simulink model "V.1.0.SystemsmModelling"  (R2020a)
settings: Solver=ode23t  StartTime=0.0  StopTime=2000  MaxStep=2000.0  RelTol=1e-3
values from neighbouring files (symbols this model uses):
  InitialTemp = 300    [Setup.m]
undefined symbols (not defined in the file or in its folder): commanded_mass_flow, compressor_time_constant, condenser_length, copper_density, environment_temperature, evaporator_length, ground_temperature, max_throat_area, max_throat_temperature, min_throat_area, min_throat_temperature, pipe_diameter, pipe_thickness, target_temperature, temperature_delta, u_sat
libraries: fl_lib x208, refrigeration_lib x90, fl_ps_legacy_lib x50, nesl_utility x45
(part 5 of 7)

== system V.1.0.SystemsmModelling/Air Conditioning System/Air Conditioner Model5/Condenser ==
  Condenser Conduction : fl_lib/Thermal/Thermal Elements/Conductive Heat Transfer  area=pi*pipe_diameter*condenser_length m^2  thickness=pipe_thickness m  th_cond=copper_conductivity W/(m*K)  T_specify=off  T_priority=High  T=0 K  T_nominal_specify=off  T_nominal_unit=K  T_nominal_value=1  Q_specify=off  Q_priority=High  Q=0 J/s  Q_nominal_specify=off  Q_nominal_unit=W  Q_nominal_value=1
  Condenser Copper : fl_lib/Thermal/Thermal Elements/Thermal Mass  mass=pi*pipe_diameter*condenser_length*pipe_thickness*copper_density kg  sp_heat=copper_specific_heat J/kg/K  T_specify=on  T_priority=High  T=environment_temperature K  T_nominal_specify=off  T_nominal_unit=K  T_nominal_value=1  Q_specify=off  Q_priority=High  Q=0 J/s  Q_nominal_specify=off  Q_nominal_unit=W  Q_nominal_value=1
  Condenser Pipe : refrigeration_lib/Pipe  L=condenser_length m  S=pi*pipe_diameter^2/4 m^2  Dh=pipe_diameter m  fs=64  La=0.1*condenser_length m  eps=15e-6 m  Re_lam=2000  Re_tur=4000  J_smooth=5 kg/m^2/s  p_0=charge_pressure MPa  T_0=-1 K  x_0=initial_quality  mdot_A_specify=off  mdot_A_priority=High  mdot_A=0 kg/s  mdot_A_nominal_specify=off  mdot_A_nominal_unit=kg/s  mdot_A_nominal_value=1  mdot_B_specify=off  mdot_B_priority=High  mdot_B=0 kg/s  mdot_B_nominal_specify=off  mdot_B_nominal_unit=kg/s  mdot_B_nominal_value=1  phi_A_specify=off  phi_A_priority=High  phi_A=0 kW  phi_A_nominal_specify=off  phi_A_nominal_unit=kW  phi_A_nominal_value=1  phi_B_specify=off  phi_B_priority=High  phi_B=0 kW  phi_B_nominal_specify=off  phi_B_nominal_unit=kW  phi_B_nominal_value=1  v_A_specify=off  v_A_priority=High  v_A=0.230606289431 m^3/kg  v_A_nominal_specify=off  v_A_nominal_unit=m^3/kg  v_A_nominal_value=1  v_B_specify=off  v_B_priority=High  v_B=0.230606289431 m^3/kg  v_B_nominal_specify=off  v_B_nominal_unit=m^3/kg  v_B_nominal_value=1  p_I_specify=off  p_I_priority=High  p_I=0.101325 MPa  p_I_nominal_specify=off  p_I_nominal_unit=MPa  p_I_nominal_value=1  u_I_specify=off  u_I_priority=High  u_I=396.921741345 kJ/kg  u_I_nominal_specify=off  u_I_nominal_unit=kJ/kg  u_I_nominal_value=1  v_I_specify=off  v_I_priority=High  v_I=0.230606289431 m^3/kg  v_I_nominal_specify=off  v_I_nominal_unit=m^3/kg  v_I_nominal_value=1  q_T_specify=off  q_T_priority=High  q_T=0 kW  q_T_nominal_specify=off  q_T_nominal_unit=kW  q_T_nominal_value=1  Ff_A_specify=off  Ff_A_priority=High  Ff_A=0 N  Ff_A_nominal_specify=off  Ff_A_nominal_unit=N  Ff_A_nominal_value=1  Ff_B_specify=off  Ff_B_priority=High  Ff_B=0 N  Ff_B_nominal_specify=off  Ff_B_nominal_unit=N  Ff_B_nominal_value=1  ev_I_specify=off  ev_I_priority=High  ev_I=1.7212095226213e+3 kJ/m^3  ev_I_nominal_specify=off  ev_I_nominal_unit=kJ/m^3  ev_I_nominal_value=1  mdot_I_specify=off  mdot_I_priority=High  mdot_I=0 kg/s  mdot_I_nominal_specify=off  mdot_I_nominal_unit=kg/s  mdot_I_nominal_value=1  Nu_I_specify=off  Nu_I_priority=High  Nu_I=0  Nu_I_nominal_specify=off  Nu_I_nominal_unit=1  Nu_I_nominal_value=1
      settings: InternalSimscapePortConfiguration="{\"Bottom\":[],\"Left\":[{\"id\":\"A\",\"label\":\"A\",\"type\":\"refrigeration.refrigeration\"},{\"id\":\"T\",\"label\":\"T\",\"type\":\"foundation.thermal.thermal\"}],\"Right\":[{\"id\":\"B\",\"label\":\"B\",\"type\":\"refrigeration.refrigeration\"}],\"Top\":[]}"
  T : PMIOPort  Side=Left
  B : PMIOPort  Port=2  Side=Left
  A : PMIOPort  Port=3  Side=Right
  connections:
  Condenser Conduction/LConn1 -- Condenser Pipe/LConn2 -- Condenser Copper/LConn1
  T/RConn1 -- Condenser Conduction/RConn1
  B/RConn1 -- Condenser Pipe/RConn1
  Condenser Pipe/LConn1 -- A/RConn1

== system V.1.0.SystemsmModelling/Air Conditioning System/Air Conditioner Model5/Control ==
  Err : Inport
  Relay : Relay  OnSwitchValue=temperature_delta  OffSwitchValue=-temperature_delta
  On : Outport
  wires:
  Err/1 -> Relay/1
  Relay/1 -> On/1

== system V.1.0.SystemsmModelling/Air Conditioning System/Air Conditioner Model5/Environment ==
  Condenser Convection : fl_lib/Thermal/Thermal Elements/Convective Heat Transfer  area=fin_area m^2  heat_tr_coeff=fin_convection_coefficient W/(m^2 * K)  T_specify=off  T_priority=High  T=0 K  T_nominal_specify=off  T_nominal_unit=K  T_nominal_value=1  Q_specify=off  Q_priority=High  Q=0 J/s  Q_nominal_specify=off  Q_nominal_unit=W  Q_nominal_value=1
  Constant : Constant  Value=environment_temperature
  Ideal Temperature Source : fl_lib/Thermal/Thermal Sources/Controlled Temperature Source
  Simulink-PS Converter : nesl_utility/Simulink-PS Converter  PhysicalDomain=network_engine_domain  SubClassName=ps_input  LeftPortType=input  RightPortType=output  PseudoPeriodic=off  Frequencies=[]  NoiseDistribution=none  NoiseParameters=[]  Unit=K  AffineConversion=off  FilteringAndDerivatives=zero  SimscapeFilterOrder=1  InputFilterTimeConstant=0.001  UdotUserProvided=1
  Thermal Reference : fl_lib/Thermal/Thermal Elements/Thermal Reference
  T : PMIOPort  Side=Left
  wires:
  Constant/1 -> Simulink-PS Converter/1
  connections:
  Condenser Convection/RConn1 -- Ideal Temperature Source/LConn1
  Condenser Convection/LConn1 -- T/RConn1
  Ideal Temperature Source/RConn1 -- Simulink-PS Converter/RConn1
  Ideal Temperature Source/RConn2 -- Thermal Reference/LConn1

== system V.1.0.SystemsmModelling/Air Conditioning System/Air Conditioner Model5/Evaporator ==
  Evaporator Conduction : fl_lib/Thermal/Thermal Elements/Conductive Heat Transfer  area=pi*pipe_diameter*evaporator_length m^2  thickness=pipe_thickness m  th_cond=copper_conductivity W/(m*K)  T_specify=off  T_priority=High  T=0 K  T_nominal_specify=off  T_nominal_unit=K  T_nominal_value=1  Q_specify=off  Q_priority=High  Q=0 J/s  Q_nominal_specify=off  Q_nominal_unit=W  Q_nominal_value=1
  Evaporator Copper : fl_lib/Thermal/Thermal Elements/Thermal Mass  mass=pi*pipe_diameter*evaporator_length*pipe_thickness*copper_density kg  sp_heat=copper_specific_heat J/kg/K  T_specify=on  T_priority=High  T=target_temperature K  T_nominal_specify=off  T_nominal_unit=K  T_nominal_value=1  Q_specify=off  Q_priority=High  Q=0 J/s  Q_nominal_specify=off  Q_nominal_unit=W  Q_nominal_value=1
  Evaporator Pipe : refrigeration_lib/Pipe  L=evaporator_length m  S=pi*pipe_diameter^2/4 m^2  Dh=pipe_diameter m  fs=64  La=0.1*evaporator_length m  eps=15e-6 m  Re_lam=2000  Re_tur=4000  J_smooth=5 kg/m^2/s  p_0=charge_pressure MPa  T_0=-1 K  x_0=initial_quality  mdot_A_specify=off  mdot_A_priority=High  mdot_A=0 kg/s  mdot_A_nominal_specify=off  mdot_A_nominal_unit=kg/s  mdot_A_nominal_value=1  mdot_B_specify=off  mdot_B_priority=High  mdot_B=0 kg/s  mdot_B_nominal_specify=off  mdot_B_nominal_unit=kg/s  mdot_B_nominal_value=1  phi_A_specify=off  phi_A_priority=High  phi_A=0 kW  phi_A_nominal_specify=off  phi_A_nominal_unit=kW  phi_A_nominal_value=1  phi_B_specify=off  phi_B_priority=High  phi_B=0 kW  phi_B_nominal_specify=off  phi_B_nominal_unit=kW  phi_B_nominal_value=1  v_A_specify=off  v_A_priority=High  v_A=0.230606289431 m^3/kg  v_A_nominal_specify=off  v_A_nominal_unit=m^3/kg  v_A_nominal_value=1  v_B_specify=off  v_B_priority=High  v_B=0.230606289431 m^3/kg  v_B_nominal_specify=off  v_B_nominal_unit=m^3/kg  v_B_nominal_value=1  p_I_specify=off  p_I_priority=High  p_I=0.101325 MPa  p_I_nominal_specify=off  p_I_nominal_unit=MPa  p_I_nominal_value=1  u_I_specify=off  u_I_priority=High  u_I=396.921741345 kJ/kg  u_I_nominal_specify=off  u_I_nominal_unit=kJ/kg  u_I_nominal_value=1  v_I_specify=off  v_I_priority=High  v_I=0.230606289431 m^3/kg  v_I_nominal_specify=off  v_I_nominal_unit=m^3/kg  v_I_nominal_value=1  q_T_specify=off  q_T_priority=High  q_T=0 kW  q_T_nominal_specify=off  q_T_nominal_unit=kW  q_T_nominal_value=1  Ff_A_specify=off  Ff_A_priority=High  Ff_A=0 N  Ff_A_nominal_specify=off  Ff_A_nominal_unit=N  Ff_A_nominal_value=1  Ff_B_specify=off  Ff_B_priority=High  Ff_B=0 N  Ff_B_nominal_specify=off  Ff_B_nominal_unit=N  Ff_B_nominal_value=1  ev_I_specify=off  ev_I_priority=High  ev_I=1.7212095226213e+3 kJ/m^3  ev_I_nominal_specify=off  ev_I_nominal_unit=kJ/m^3  ev_I_nominal_value=1  mdot_I_specify=off  mdot_I_priority=High  mdot_I=0 kg/s  mdot_I_nominal_specify=off  mdot_I_nominal_unit=kg/s  mdot_I_nominal_value=1  Nu_I_specify=off  Nu_I_priority=High  Nu_I=0  Nu_I_nominal_specify=off  Nu_I_nominal_unit=1  Nu_I_nominal_value=1
      settings: InternalSimscapePortConfiguration="{\"Bottom\":[],\"Left\":[{\"id\":\"A\",\"label\":\"A\",\"type\":\"refrigeration.refrigeration\"},{\"id\":\"T\",\"label\":\"T\",\"type\":\"foundation.thermal.thermal\"}],\"Right\":[{\"id\":\"B\",\"label\":\"B\",\"type\":\"refrigeration.refrigeration\"}],\"Top\":[]}"
  A : PMIOPort  Side=Left
  B : PMIOPort  Port=2  Side=Right
  T : PMIOPort  Port=3  Side=Right
  connections:
  Evaporator Conduction/RConn1 -- T/RConn1
  Evaporator Copper/LConn1 -- Evaporator Pipe/LConn2 -- Evaporator Conduction/LConn1
  Evaporator Pipe/RConn1 -- B/RConn1
  Evaporator Pipe/LConn1 -- A/RConn1

== system V.1.0.SystemsmModelling/Air Conditioning System/Air Conditioner Model5/Expansion Valve ==
  Controlled Local Restriction : refrigeration_lib/Controlled Local Restriction  Cd=0.7  L=0.1 m  S=pi*pipe_diameter^2/4 m^2
      settings: InternalSimscapePortConfiguration="{\"Bottom\":[],\"Left\":[{\"id\":\"A\",\"label\":\"A\",\"type\":\"refrigeration.refrigeration\"},{\"id\":\"Sr\",\"label\":\"S\",\"type\":\"input\"}],\"Right\":[{\"id\":\"B\",\"label\":\"B\",\"type\":\"refrigeration.refrigeration\"}],\"Top\":[]}"
  Cycle Sensor 4 : Subsystem
  Mass Flow Sensor : Subsystem
  Valve Control : Subsystem
  A : PMIOPort  Side=Left
  B : PMIOPort  Port=2  Side=Right
  connections:
  B/RConn1 -- Cycle Sensor 4/LConn1 -- Mass Flow Sensor/RConn1
  Controlled Local Restriction/LConn1 -- A/RConn1
  Controlled Local Restriction/RConn1 -- Mass Flow Sensor/LConn1
  Controlled Local Restriction/LConn2 -- Valve Control/LConn1
  Cycle Sensor 4/RConn1 -- Valve Control/RConn1

== system V.1.0.SystemsmModelling/Air Conditioning System/Air Conditioner Model5/Plot Properties ==

== system V.1.0.SystemsmModelling/Air Conditioning System/Air Conditioner Model5/Refrigerator Compartment ==
  Environment Temperature : Subsystem
  Evaporator Convection : fl_lib/Thermal/Thermal Elements/Convective Heat Transfer  area=interior_surface_area m^2  heat_tr_coeff=natural_convection_coefficient W/(m^2 * K)  T_specify=off  T_priority=High  T=0 K  T_nominal_specify=off  T_nominal_unit=K  T_nominal_value=1  Q_specify=off  Q_priority=High  Q=0 J/s  Q_nominal_specify=off  Q_nominal_unit=W  Q_nominal_value=1
  Heat Flow Sensor : Subsystem
  Polyurethane Foam Conduction : fl_lib/Thermal/Thermal Elements/Conductive Heat Transfer  area=interior_surface_area m^2  thickness=foam_thickness m  th_cond=foam_conductivity W/(m*K)  T_specify=off  T_priority=High  T=0 K  T_nominal_specify=off  T_nominal_unit=K  T_nominal_value=1  Q_specify=off  Q_priority=High  Q=0 J/s  Q_nominal_specify=off  Q_nominal_unit=W  Q_nominal_value=1
  Refrigerator Convection Exterior : fl_lib/Thermal/Thermal Elements/Convective Heat Transfer  area=exterior_surface_area m^2  heat_tr_coeff=natural_convection_coefficient W/(m^2 * K)  T_specify=off  T_priority=High  T=0 K  T_nominal_specify=off  T_nominal_unit=K  T_nominal_value=1  Q_specify=off  Q_priority=High  Q=0 J/s  Q_nominal_specify=off  Q_nominal_unit=W  Q_nominal_value=1
  Refrigerator Convection Interior : fl_lib/Thermal/Thermal Elements/Convective Heat Transfer  area=interior_surface_area m^2  heat_tr_coeff=natural_convection_coefficient W/(m^2 * K)  T_specify=off  T_priority=High  T=0 K  T_nominal_specify=off  T_nominal_unit=K  T_nominal_value=1  Q_specify=off  Q_priority=High  Q=0 J/s  Q_nominal_specify=off  Q_nominal_unit=W  Q_nominal_value=1
  Temperature Sensor : Subsystem
  T : PMIOPort  Side=Left
  Air : PMIOPort  Port=2  Side=Left
  S : Outport
  wires:
  Temperature Sensor/1(T) -> S/1
  connections:
  Evaporator Convection/LConn1 -- Heat Flow Sensor/RConn1
  T/RConn1 -- Heat Flow Sensor/LConn1
  Refrigerator Convection Exterior/RConn1 -- Environment Temperature/LConn1
  Refrigerator Convection Interior/LConn1 -- Evaporator Convection/RConn1 -- Temperature Sensor/LConn1 -- Air/RConn1
  Refrigerator Convection Interior/RConn1 -- Polyurethane Foam Conduction/LConn1
  Polyurethane Foam Conduction/RConn1 -- Refrigerator Convection Exterior/LConn1

== system V.1.0.SystemsmModelling/Air Conditioning System/Air Conditioner Model6/Compressor ==
  On : Inport
  Commanded Mass Flow Rate : Gain  Gain=commanded_mass_flow
  Compressor Lag : TransferFcn  Numerator=[(9/compressor_time_constant)^2]  Denominator=[1, 2*(9/compressor_time_constant), (9/compressor_time_constant)^2]
  Controlled Mass Flow Rate Source : refrigeration_lib/Controlled Mass Flow Rate Source  S=pi*pipe_diameter^2/4 m^2  L=0.1 m  mdot_specify=off  mdot_priority=High  mdot=0 kg/s  mdot_nominal_specify=off  mdot_nominal_unit=kg/s  mdot_nominal_value=1  phi_A_specify=off  phi_A_priority=High  phi_A=0 kW  phi_A_nominal_specify=off  phi_A_nominal_unit=kW  phi_A_nominal_value=1  phi_B_specify=off  phi_B_priority=High  phi_B=0 kW  phi_B_nominal_specify=off  phi_B_nominal_unit=kW  phi_B_nominal_value=1  u_AI_specify=off  u_AI_priority=High  u_AI=396.921741345 kJ/kg  u_AI_nominal_specify=off  u_AI_nominal_unit=kJ/kg  u_AI_nominal_value=1  v_A_specify=off  v_A_priority=High  v_A=0.230606289431 m^3/kg  v_A_nominal_specify=off  v_A_nominal_unit=m^3/kg  v_A_nominal_value=1  u_BI_specify=off  u_BI_priority=High  u_BI=396.921741345 kJ/kg  u_BI_nominal_specify=off  u_BI_nominal_unit=kJ/kg  u_BI_nominal_value=1  v_B_specify=off  v_B_priority=High  v_B=0.230606289431 m^3/kg  v_B_nominal_specify=off  v_B_nominal_unit=m^3/kg  v_B_nominal_value=1  u_2_specify=off  u_2_priority=High  u_2=396.921741345 kJ/kg  u_2_nominal_specify=off  u_2_nominal_unit=kJ/kg  u_2_nominal_value=1  u_3_specify=off  u_3_priority=High  u_3=396.921741345 kJ/kg  u_3_nominal_specify=off  u_3_nominal_unit=kJ/kg  u_3_nominal_value=1
      settings: InternalSimscapePortConfiguration="{\"Bottom\":[],\"Left\":[{\"id\":\"A\",\"label\":\"A\",\"type\":\"refrigeration.refrigeration\"},{\"id\":\"M\",\"label\":\"M\",\"type\":\"input\"}],\"Right\":[{\"id\":\"B\",\"label\":\"B\",\"type\":\"refrigeration.refrigeration\"},{\"id\":\"W\",\"label\":\"W\",\"type\":\"output\"}],\"Top\":[]}"
  Simulink-PS Converter : nesl_utility/Simulink-PS Converter  PhysicalDomain=network_engine_domain  SubClassName=ps_input  LeftPortType=input  RightPortType=output  PseudoPeriodic=off  Frequencies=[]  NoiseDistribution=none  NoiseParameters=[]  Unit=kg/s  AffineConversion=off  FilteringAndDerivatives=zero  SimscapeFilterOrder=1  InputFilterTimeConstant=0.001  UdotUserProvided=1
  B : PMIOPort  Side=Right
  A : PMIOPort  Port=2  Side=Left
  wires:
  Compressor Lag/1 -> Simulink-PS Converter/1
  Commanded Mass Flow Rate/1 -> Compressor Lag/1
  On/1 -> Commanded Mass Flow Rate/1
  connections:
  Controlled Mass Flow Rate Source/RConn1 -- B/RConn1
  Controlled Mass Flow Rate Source/LConn2 -- Simulink-PS Converter/RConn1
  A/RConn1 -- Controlled Mass Flow Rate Source/LConn1

== system V.1.0.SystemsmModelling/Air Conditioning System/Air Conditioner Model6/Condenser ==
  Condenser Conduction : fl_lib/Thermal/Thermal Elements/Conductive Heat Transfer  area=pi*pipe_diameter*condenser_length m^2  thickness=pipe_thickness m  th_cond=copper_conductivity W/(m*K)  T_specify=off  T_priority=High  T=0 K  T_nominal_specify=off  T_nominal_unit=K  T_nominal_value=1  Q_specify=off  Q_priority=High  Q=0 J/s  Q_nominal_specify=off  Q_nominal_unit=W  Q_nominal_value=1
  Condenser Copper : fl_lib/Thermal/Thermal Elements/Thermal Mass  mass=pi*pipe_diameter*condenser_length*pipe_thickness*copper_density kg  sp_heat=copper_specific_heat J/kg/K  T_specify=on  T_priority=High  T=environment_temperature K  T_nominal_specify=off  T_nominal_unit=K  T_nominal_value=1  Q_specify=off  Q_priority=High  Q=0 J/s  Q_nominal_specify=off  Q_nominal_unit=W  Q_nominal_value=1
  Condenser Pipe : refrigeration_lib/Pipe  L=condenser_length m  S=pi*pipe_diameter^2/4 m^2  Dh=pipe_diameter m  fs=64  La=0.1*condenser_length m  eps=15e-6 m  Re_lam=2000  Re_tur=4000  J_smooth=5 kg/m^2/s  p_0=charge_pressure MPa  T_0=-1 K  x_0=initial_quality  mdot_A_specify=off  mdot_A_priority=High  mdot_A=0 kg/s  mdot_A_nominal_specify=off  mdot_A_nominal_unit=kg/s  mdot_A_nominal_value=1  mdot_B_specify=off  mdot_B_priority=High  mdot_B=0 kg/s  mdot_B_nominal_specify=off  mdot_B_nominal_unit=kg/s  mdot_B_nominal_value=1  phi_A_specify=off  phi_A_priority=High  phi_A=0 kW  phi_A_nominal_specify=off  phi_A_nominal_unit=kW  phi_A_nominal_value=1  phi_B_specify=off  phi_B_priority=High  phi_B=0 kW  phi_B_nominal_specify=off  phi_B_nominal_unit=kW  phi_B_nominal_value=1  v_A_specify=off  v_A_priority=High  v_A=0.230606289431 m^3/kg  v_A_nominal_specify=off  v_A_nominal_unit=m^3/kg  v_A_nominal_value=1  v_B_specify=off  v_B_priority=High  v_B=0.230606289431 m^3/kg  v_B_nominal_specify=off  v_B_nominal_unit=m^3/kg  v_B_nominal_value=1  p_I_specify=off  p_I_priority=High  p_I=0.101325 MPa  p_I_nominal_specify=off  p_I_nominal_unit=MPa  p_I_nominal_value=1  u_I_specify=off  u_I_priority=High  u_I=396.921741345 kJ/kg  u_I_nominal_specify=off  u_I_nominal_unit=kJ/kg  u_I_nominal_value=1  v_I_specify=off  v_I_priority=High  v_I=0.230606289431 m^3/kg  v_I_nominal_specify=off  v_I_nominal_unit=m^3/kg  v_I_nominal_value=1  q_T_specify=off  q_T_priority=High  q_T=0 kW  q_T_nominal_specify=off  q_T_nominal_unit=kW  q_T_nominal_value=1  Ff_A_specify=off  Ff_A_priority=High  Ff_A=0 N  Ff_A_nominal_specify=off  Ff_A_nominal_unit=N  Ff_A_nominal_value=1  Ff_B_specify=off  Ff_B_priority=High  Ff_B=0 N  Ff_B_nominal_specify=off  Ff_B_nominal_unit=N  Ff_B_nominal_value=1  ev_I_specify=off  ev_I_priority=High  ev_I=1.7212095226213e+3 kJ/m^3  ev_I_nominal_specify=off  ev_I_nominal_unit=kJ/m^3  ev_I_nominal_value=1  mdot_I_specify=off  mdot_I_priority=High  mdot_I=0 kg/s  mdot_I_nominal_specify=off  mdot_I_nominal_unit=kg/s  mdot_I_nominal_value=1  Nu_I_specify=off  Nu_I_priority=High  Nu_I=0  Nu_I_nominal_specify=off  Nu_I_nominal_unit=1  Nu_I_nominal_value=1
      settings: InternalSimscapePortConfiguration="{\"Bottom\":[],\"Left\":[{\"id\":\"A\",\"label\":\"A\",\"type\":\"refrigeration.refrigeration\"},{\"id\":\"T\",\"label\":\"T\",\"type\":\"foundation.thermal.thermal\"}],\"Right\":[{\"id\":\"B\",\"label\":\"B\",\"type\":\"refrigeration.refrigeration\"}],\"Top\":[]}"
  T : PMIOPort  Side=Left
  B : PMIOPort  Port=2  Side=Left
  A : PMIOPort  Port=3  Side=Right
  connections:
  Condenser Conduction/LConn1 -- Condenser Pipe/LConn2 -- Condenser Copper/LConn1
  T/RConn1 -- Condenser Conduction/RConn1
  B/RConn1 -- Condenser Pipe/RConn1
  Condenser Pipe/LConn1 -- A/RConn1

== system V.1.0.SystemsmModelling/Air Conditioning System/Air Conditioner Model6/Control ==
  Err : Inport
  Relay : Relay  OnSwitchValue=temperature_delta  OffSwitchValue=-temperature_delta
  On : Outport
  wires:
  Err/1 -> Relay/1
  Relay/1 -> On/1

== system V.1.0.SystemsmModelling/Air Conditioning System/Air Conditioner Model6/Environment ==
  Condenser Convection : fl_lib/Thermal/Thermal Elements/Convective Heat Transfer  area=fin_area m^2  heat_tr_coeff=fin_convection_coefficient W/(m^2 * K)  T_specify=off  T_priority=High  T=0 K  T_nominal_specify=off  T_nominal_unit=K  T_nominal_value=1  Q_specify=off  Q_priority=High  Q=0 J/s  Q_nominal_specify=off  Q_nominal_unit=W  Q_nominal_value=1
  Constant : Constant  Value=environment_temperature
  Ideal Temperature Source : fl_lib/Thermal/Thermal Sources/Controlled Temperature Source
  Simulink-PS Converter : nesl_utility/Simulink-PS Converter  PhysicalDomain=network_engine_domain  SubClassName=ps_input  LeftPortType=input  RightPortType=output  PseudoPeriodic=off  Frequencies=[]  NoiseDistribution=none  NoiseParameters=[]  Unit=K  AffineConversion=off  FilteringAndDerivatives=zero  SimscapeFilterOrder=1  InputFilterTimeConstant=0.001  UdotUserProvided=1
  Thermal Reference : fl_lib/Thermal/Thermal Elements/Thermal Reference
  T : PMIOPort  Side=Left
  wires:
  Constant/1 -> Simulink-PS Converter/1
  connections:
  Condenser Convection/RConn1 -- Ideal Temperature Source/LConn1
  Condenser Convection/LConn1 -- T/RConn1
  Ideal Temperature Source/RConn1 -- Simulink-PS Converter/RConn1
  Ideal Temperature Source/RConn2 -- Thermal Reference/LConn1

== system V.1.0.SystemsmModelling/Air Conditioning System/Air Conditioner Model6/Evaporator ==
  Evaporator Conduction : fl_lib/Thermal/Thermal Elements/Conductive Heat Transfer  area=pi*pipe_diameter*evaporator_length m^2  thickness=pipe_thickness m  th_cond=copper_conductivity W/(m*K)  T_specify=off  T_priority=High  T=0 K  T_nominal_specify=off  T_nominal_unit=K  T_nominal_value=1  Q_specify=off  Q_priority=High  Q=0 J/s  Q_nominal_specify=off  Q_nominal_unit=W  Q_nominal_value=1
  Evaporator Copper : fl_lib/Thermal/Thermal Elements/Thermal Mass  mass=pi*pipe_diameter*evaporator_length*pipe_thickness*copper_density kg  sp_heat=copper_specific_heat J/kg/K  T_specify=on  T_priority=High  T=target_temperature K  T_nominal_specify=off  T_nominal_unit=K  T_nominal_value=1  Q_specify=off  Q_priority=High  Q=0 J/s  Q_nominal_specify=off  Q_nominal_unit=W  Q_nominal_value=1
  Evaporator Pipe : refrigeration_lib/Pipe  L=evaporator_length m  S=pi*pipe_diameter^2/4 m^2  Dh=pipe_diameter m  fs=64  La=0.1*evaporator_length m  eps=15e-6 m  Re_lam=2000  Re_tur=4000  J_smooth=5 kg/m^2/s  p_0=charge_pressure MPa  T_0=-1 K  x_0=initial_quality  mdot_A_specify=off  mdot_A_priority=High  mdot_A=0 kg/s  mdot_A_nominal_specify=off  mdot_A_nominal_unit=kg/s  mdot_A_nominal_value=1  mdot_B_specify=off  mdot_B_priority=High  mdot_B=0 kg/s  mdot_B_nominal_specify=off  mdot_B_nominal_unit=kg/s  mdot_B_nominal_value=1  phi_A_specify=off  phi_A_priority=High  phi_A=0 kW  phi_A_nominal_specify=off  phi_A_nominal_unit=kW  phi_A_nominal_value=1  phi_B_specify=off  phi_B_priority=High  phi_B=0 kW  phi_B_nominal_specify=off  phi_B_nominal_unit=kW  phi_B_nominal_value=1  v_A_specify=off  v_A_priority=High  v_A=0.230606289431 m^3/kg  v_A_nominal_specify=off  v_A_nominal_unit=m^3/kg  v_A_nominal_value=1  v_B_specify=off  v_B_priority=High  v_B=0.230606289431 m^3/kg  v_B_nominal_specify=off  v_B_nominal_unit=m^3/kg  v_B_nominal_value=1  p_I_specify=off  p_I_priority=High  p_I=0.101325 MPa  p_I_nominal_specify=off  p_I_nominal_unit=MPa  p_I_nominal_value=1  u_I_specify=off  u_I_priority=High  u_I=396.921741345 kJ/kg  u_I_nominal_specify=off  u_I_nominal_unit=kJ/kg  u_I_nominal_value=1  v_I_specify=off  v_I_priority=High  v_I=0.230606289431 m^3/kg  v_I_nominal_specify=off  v_I_nominal_unit=m^3/kg  v_I_nominal_value=1  q_T_specify=off  q_T_priority=High  q_T=0 kW  q_T_nominal_specify=off  q_T_nominal_unit=kW  q_T_nominal_value=1  Ff_A_specify=off  Ff_A_priority=High  Ff_A=0 N  Ff_A_nominal_specify=off  Ff_A_nominal_unit=N  Ff_A_nominal_value=1  Ff_B_specify=off  Ff_B_priority=High  Ff_B=0 N  Ff_B_nominal_specify=off  Ff_B_nominal_unit=N  Ff_B_nominal_value=1  ev_I_specify=off  ev_I_priority=High  ev_I=1.7212095226213e+3 kJ/m^3  ev_I_nominal_specify=off  ev_I_nominal_unit=kJ/m^3  ev_I_nominal_value=1  mdot_I_specify=off  mdot_I_priority=High  mdot_I=0 kg/s  mdot_I_nominal_specify=off  mdot_I_nominal_unit=kg/s  mdot_I_nominal_value=1  Nu_I_specify=off  Nu_I_priority=High  Nu_I=0  Nu_I_nominal_specify=off  Nu_I_nominal_unit=1  Nu_I_nominal_value=1
      settings: InternalSimscapePortConfiguration="{\"Bottom\":[],\"Left\":[{\"id\":\"A\",\"label\":\"A\",\"type\":\"refrigeration.refrigeration\"},{\"id\":\"T\",\"label\":\"T\",\"type\":\"foundation.thermal.thermal\"}],\"Right\":[{\"id\":\"B\",\"label\":\"B\",\"type\":\"refrigeration.refrigeration\"}],\"Top\":[]}"
  A : PMIOPort  Side=Left
  B : PMIOPort  Port=2  Side=Right
  T : PMIOPort  Port=3  Side=Right
  connections:
  Evaporator Conduction/RConn1 -- T/RConn1
  Evaporator Copper/LConn1 -- Evaporator Pipe/LConn2 -- Evaporator Conduction/LConn1
  Evaporator Pipe/RConn1 -- B/RConn1
  Evaporator Pipe/LConn1 -- A/RConn1

== system V.1.0.SystemsmModelling/Air Conditioning System/Air Conditioner Model6/Expansion Valve ==
  Controlled Local Restriction : refrigeration_lib/Controlled Local Restriction  Cd=0.7  L=0.1 m  S=pi*pipe_diameter^2/4 m^2
      settings: InternalSimscapePortConfiguration="{\"Bottom\":[],\"Left\":[{\"id\":\"A\",\"label\":\"A\",\"type\":\"refrigeration.refrigeration\"},{\"id\":\"Sr\",\"label\":\"S\",\"type\":\"input\"}],\"Right\":[{\"id\":\"B\",\"label\":\"B\",\"type\":\"refrigeration.refrigeration\"}],\"Top\":[]}"
  Cycle Sensor 4 : Subsystem
  Mass Flow Sensor : Subsystem
  Valve Control : Subsystem
  A : PMIOPort  Side=Left
  B : PMIOPort  Port=2  Side=Right
  connections:
  B/RConn1 -- Cycle Sensor 4/LConn1 -- Mass Flow Sensor/RConn1
  Controlled Local Restriction/LConn1 -- A/RConn1
  Controlled Local Restriction/RConn1 -- Mass Flow Sensor/LConn1
  Controlled Local Restriction/LConn2 -- Valve Control/LConn1
  Cycle Sensor 4/RConn1 -- Valve Control/RConn1

== system V.1.0.SystemsmModelling/Air Conditioning System/Air Conditioner Model6/Plot Properties ==

== system V.1.0.SystemsmModelling/Air Conditioning System/Air Conditioner Model6/Refrigerator Compartment ==
  Environment Temperature : Subsystem
  Evaporator Convection : fl_lib/Thermal/Thermal Elements/Convective Heat Transfer  area=interior_surface_area m^2  heat_tr_coeff=natural_convection_coefficient W/(m^2 * K)  T_specify=off  T_priority=High  T=0 K  T_nominal_specify=off  T_nominal_unit=K  T_nominal_value=1  Q_specify=off  Q_priority=High  Q=0 J/s  Q_nominal_specify=off  Q_nominal_unit=W  Q_nominal_value=1
  Heat Flow Sensor : Subsystem
  Polyurethane Foam Conduction : fl_lib/Thermal/Thermal Elements/Conductive Heat Transfer  area=interior_surface_area m^2  thickness=foam_thickness m  th_cond=foam_conductivity W/(m*K)  T_specify=off  T_priority=High  T=0 K  T_nominal_specify=off  T_nominal_unit=K  T_nominal_value=1  Q_specify=off  Q_priority=High  Q=0 J/s  Q_nominal_specify=off  Q_nominal_unit=W  Q_nominal_value=1
  Refrigerator Convection Exterior : fl_lib/Thermal/Thermal Elements/Convective Heat Transfer  area=exterior_surface_area m^2  heat_tr_coeff=natural_convection_coefficient W/(m^2 * K)  T_specify=off  T_priority=High  T=0 K  T_nominal_specify=off  T_nominal_unit=K  T_nominal_value=1  Q_specify=off  Q_priority=High  Q=0 J/s  Q_nominal_specify=off  Q_nominal_unit=W  Q_nominal_value=1
  Refrigerator Convection Interior : fl_lib/Thermal/Thermal Elements/Convective Heat Transfer  area=interior_surface_area m^2  heat_tr_coeff=natural_convection_coefficient W/(m^2 * K)  T_specify=off  T_priority=High  T=0 K  T_nominal_specify=off  T_nominal_unit=K  T_nominal_value=1  Q_specify=off  Q_priority=High  Q=0 J/s  Q_nominal_specify=off  Q_nominal_unit=W  Q_nominal_value=1
  Temperature Sensor : Subsystem
  T : PMIOPort  Side=Left
  Air : PMIOPort  Port=2  Side=Left
  S : Outport
  wires:
  Temperature Sensor/1(T) -> S/1
  connections:
  Evaporator Convection/LConn1 -- Heat Flow Sensor/RConn1
  T/RConn1 -- Heat Flow Sensor/LConn1
  Refrigerator Convection Exterior/RConn1 -- Environment Temperature/LConn1
  Refrigerator Convection Interior/LConn1 -- Evaporator Convection/RConn1 -- Temperature Sensor/LConn1 -- Air/RConn1
  Refrigerator Convection Interior/RConn1 -- Polyurethane Foam Conduction/LConn1
  Polyurethane Foam Conduction/RConn1 -- Refrigerator Convection Exterior/LConn1

== system V.1.0.SystemsmModelling/Air Conditioning System/Air Conditioner Model7/Compressor ==
  On : Inport
  Commanded Mass Flow Rate : Gain  Gain=commanded_mass_flow
  Compressor Lag : TransferFcn  Numerator=[(9/compressor_time_constant)^2]  Denominator=[1, 2*(9/compressor_time_constant), (9/compressor_time_constant)^2]
  Controlled Mass Flow Rate Source : refrigeration_lib/Controlled Mass Flow Rate Source  S=pi*pipe_diameter^2/4 m^2  L=0.1 m  mdot_specify=off  mdot_priority=High  mdot=0 kg/s  mdot_nominal_specify=off  mdot_nominal_unit=kg/s  mdot_nominal_value=1  phi_A_specify=off  phi_A_priority=High  phi_A=0 kW  phi_A_nominal_specify=off  phi_A_nominal_unit=kW  phi_A_nominal_value=1  phi_B_specify=off  phi_B_priority=High  phi_B=0 kW  phi_B_nominal_specify=off  phi_B_nominal_unit=kW  phi_B_nominal_value=1  u_AI_specify=off  u_AI_priority=High  u_AI=396.921741345 kJ/kg  u_AI_nominal_specify=off  u_AI_nominal_unit=kJ/kg  u_AI_nominal_value=1  v_A_specify=off  v_A_priority=High  v_A=0.230606289431 m^3/kg  v_A_nominal_specify=off  v_A_nominal_unit=m^3/kg  v_A_nominal_value=1  u_BI_specify=off  u_BI_priority=High  u_BI=396.921741345 kJ/kg  u_BI_nominal_specify=off  u_BI_nominal_unit=kJ/kg  u_BI_nominal_value=1  v_B_specify=off  v_B_priority=High  v_B=0.230606289431 m^3/kg  v_B_nominal_specify=off  v_B_nominal_unit=m^3/kg  v_B_nominal_value=1  u_2_specify=off  u_2_priority=High  u_2=396.921741345 kJ/kg  u_2_nominal_specify=off  u_2_nominal_unit=kJ/kg  u_2_nominal_value=1  u_3_specify=off  u_3_priority=High  u_3=396.921741345 kJ/kg  u_3_nominal_specify=off  u_3_nominal_unit=kJ/kg  u_3_nominal_value=1
      settings: InternalSimscapePortConfiguration="{\"Bottom\":[],\"Left\":[{\"id\":\"A\",\"label\":\"A\",\"type\":\"refrigeration.refrigeration\"},{\"id\":\"M\",\"label\":\"M\",\"type\":\"input\"}],\"Right\":[{\"id\":\"B\",\"label\":\"B\",\"type\":\"refrigeration.refrigeration\"},{\"id\":\"W\",\"label\":\"W\",\"type\":\"output\"}],\"Top\":[]}"
  Simulink-PS Converter : nesl_utility/Simulink-PS Converter  PhysicalDomain=network_engine_domain  SubClassName=ps_input  LeftPortType=input  RightPortType=output  PseudoPeriodic=off  Frequencies=[]  NoiseDistribution=none  NoiseParameters=[]  Unit=kg/s  AffineConversion=off  FilteringAndDerivatives=zero  SimscapeFilterOrder=1  InputFilterTimeConstant=0.001  UdotUserProvided=1
  B : PMIOPort  Side=Right
  A : PMIOPort  Port=2  Side=Left
  wires:
  Compressor Lag/1 -> Simulink-PS Converter/1
  Commanded Mass Flow Rate/1 -> Compressor Lag/1
  On/1 -> Commanded Mass Flow Rate/1
  connections:
  Controlled Mass Flow Rate Source/RConn1 -- B/RConn1
  Controlled Mass Flow Rate Source/LConn2 -- Simulink-PS Converter/RConn1
  A/RConn1 -- Controlled Mass Flow Rate Source/LConn1

== system V.1.0.SystemsmModelling/Air Conditioning System/Air Conditioner Model7/Condenser ==
  Condenser Conduction : fl_lib/Thermal/Thermal Elements/Conductive Heat Transfer  area=pi*pipe_diameter*condenser_length m^2  thickness=pipe_thickness m  th_cond=copper_conductivity W/(m*K)  T_specify=off  T_priority=High  T=0 K  T_nominal_specify=off  T_nominal_unit=K  T_nominal_value=1  Q_specify=off  Q_priority=High  Q=0 J/s  Q_nominal_specify=off  Q_nominal_unit=W  Q_nominal_value=1
  Condenser Copper : fl_lib/Thermal/Thermal Elements/Thermal Mass  mass=pi*pipe_diameter*condenser_length*pipe_thickness*copper_density kg  sp_heat=copper_specific_heat J/kg/K  T_specify=on  T_priority=High  T=environment_temperature K  T_nominal_specify=off  T_nominal_unit=K  T_nominal_value=1  Q_specify=off  Q_priority=High  Q=0 J/s  Q_nominal_specify=off  Q_nominal_unit=W  Q_nominal_value=1
  Condenser Pipe : refrigeration_lib/Pipe  L=condenser_length m  S=pi*pipe_diameter^2/4 m^2  Dh=pipe_diameter m  fs=64  La=0.1*condenser_length m  eps=15e-6 m  Re_lam=2000  Re_tur=4000  J_smooth=5 kg/m^2/s  p_0=charge_pressure MPa  T_0=-1 K  x_0=initial_quality  mdot_A_specify=off  mdot_A_priority=High  mdot_A=0 kg/s  mdot_A_nominal_specify=off  mdot_A_nominal_unit=kg/s  mdot_A_nominal_value=1  mdot_B_specify=off  mdot_B_priority=High  mdot_B=0 kg/s  mdot_B_nominal_specify=off  mdot_B_nominal_unit=kg/s  mdot_B_nominal_value=1  phi_A_specify=off  phi_A_priority=High  phi_A=0 kW  phi_A_nominal_specify=off  phi_A_nominal_unit=kW  phi_A_nominal_value=1  phi_B_specify=off  phi_B_priority=High  phi_B=0 kW  phi_B_nominal_specify=off  phi_B_nominal_unit=kW  phi_B_nominal_value=1  v_A_specify=off  v_A_priority=High  v_A=0.230606289431 m^3/kg  v_A_nominal_specify=off  v_A_nominal_unit=m^3/kg  v_A_nominal_value=1  v_B_specify=off  v_B_priority=High  v_B=0.230606289431 m^3/kg  v_B_nominal_specify=off  v_B_nominal_unit=m^3/kg  v_B_nominal_value=1  p_I_specify=off  p_I_priority=High  p_I=0.101325 MPa  p_I_nominal_specify=off  p_I_nominal_unit=MPa  p_I_nominal_value=1  u_I_specify=off  u_I_priority=High  u_I=396.921741345 kJ/kg  u_I_nominal_specify=off  u_I_nominal_unit=kJ/kg  u_I_nominal_value=1  v_I_specify=off  v_I_priority=High  v_I=0.230606289431 m^3/kg  v_I_nominal_specify=off  v_I_nominal_unit=m^3/kg  v_I_nominal_value=1  q_T_specify=off  q_T_priority=High  q_T=0 kW  q_T_nominal_specify=off  q_T_nominal_unit=kW  q_T_nominal_value=1  Ff_A_specify=off  Ff_A_priority=High  Ff_A=0 N  Ff_A_nominal_specify=off  Ff_A_nominal_unit=N  Ff_A_nominal_value=1  Ff_B_specify=off  Ff_B_priority=High  Ff_B=0 N  Ff_B_nominal_specify=off  Ff_B_nominal_unit=N  Ff_B_nominal_value=1  ev_I_specify=off  ev_I_priority=High  ev_I=1.7212095226213e+3 kJ/m^3  ev_I_nominal_specify=off  ev_I_nominal_unit=kJ/m^3  ev_I_nominal_value=1  mdot_I_specify=off  mdot_I_priority=High  mdot_I=0 kg/s  mdot_I_nominal_specify=off  mdot_I_nominal_unit=kg/s  mdot_I_nominal_value=1  Nu_I_specify=off  Nu_I_priority=High  Nu_I=0  Nu_I_nominal_specify=off  Nu_I_nominal_unit=1  Nu_I_nominal_value=1
      settings: InternalSimscapePortConfiguration="{\"Bottom\":[],\"Left\":[{\"id\":\"A\",\"label\":\"A\",\"type\":\"refrigeration.refrigeration\"},{\"id\":\"T\",\"label\":\"T\",\"type\":\"foundation.thermal.thermal\"}],\"Right\":[{\"id\":\"B\",\"label\":\"B\",\"type\":\"refrigeration.refrigeration\"}],\"Top\":[]}"
  T : PMIOPort  Side=Left
  B : PMIOPort  Port=2  Side=Left
  A : PMIOPort  Port=3  Side=Right
  connections:
  Condenser Conduction/LConn1 -- Condenser Pipe/LConn2 -- Condenser Copper/LConn1
  T/RConn1 -- Condenser Conduction/RConn1
  B/RConn1 -- Condenser Pipe/RConn1
  Condenser Pipe/LConn1 -- A/RConn1

== system V.1.0.SystemsmModelling/Air Conditioning System/Air Conditioner Model7/Control ==
  Err : Inport
  Relay : Relay  OnSwitchValue=temperature_delta  OffSwitchValue=-temperature_delta
  On : Outport
  wires:
  Err/1 -> Relay/1
  Relay/1 -> On/1

== system V.1.0.SystemsmModelling/Air Conditioning System/Air Conditioner Model7/Environment ==
  Condenser Convection : fl_lib/Thermal/Thermal Elements/Convective Heat Transfer  area=fin_area m^2  heat_tr_coeff=fin_convection_coefficient W/(m^2 * K)  T_specify=off  T_priority=High  T=0 K  T_nominal_specify=off  T_nominal_unit=K  T_nominal_value=1  Q_specify=off  Q_priority=High  Q=0 J/s  Q_nominal_specify=off  Q_nominal_unit=W  Q_nominal_value=1
  Constant : Constant  Value=environment_temperature
  Ideal Temperature Source : fl_lib/Thermal/Thermal Sources/Controlled Temperature Source
  Simulink-PS Converter : nesl_utility/Simulink-PS Converter  PhysicalDomain=network_engine_domain  SubClassName=ps_input  LeftPortType=input  RightPortType=output  PseudoPeriodic=off  Frequencies=[]  NoiseDistribution=none  NoiseParameters=[]  Unit=K  AffineConversion=off  FilteringAndDerivatives=zero  SimscapeFilterOrder=1  InputFilterTimeConstant=0.001  UdotUserProvided=1
  Thermal Reference : fl_lib/Thermal/Thermal Elements/Thermal Reference
  T : PMIOPort  Side=Left
  wires:
  Constant/1 -> Simulink-PS Converter/1
  connections:
  Condenser Convection/RConn1 -- Ideal Temperature Source/LConn1
  Condenser Convection/LConn1 -- T/RConn1
  Ideal Temperature Source/RConn1 -- Simulink-PS Converter/RConn1
  Ideal Temperature Source/RConn2 -- Thermal Reference/LConn1

== system V.1.0.SystemsmModelling/Air Conditioning System/Air Conditioner Model7/Evaporator ==
  Evaporator Conduction : fl_lib/Thermal/Thermal Elements/Conductive Heat Transfer  area=pi*pipe_diameter*evaporator_length m^2  thickness=pipe_thickness m  th_cond=copper_conductivity W/(m*K)  T_specify=off  T_priority=High  T=0 K  T_nominal_specify=off  T_nominal_unit=K  T_nominal_value=1  Q_specify=off  Q_priority=High  Q=0 J/s  Q_nominal_specify=off  Q_nominal_unit=W  Q_nominal_value=1
  Evaporator Copper : fl_lib/Thermal/Thermal Elements/Thermal Mass  mass=pi*pipe_diameter*evaporator_length*pipe_thickness*copper_density kg  sp_heat=copper_specific_heat J/kg/K  T_specify=on  T_priority=High  T=target_temperature K  T_nominal_specify=off  T_nominal_unit=K  T_nominal_value=1  Q_specify=off  Q_priority=High  Q=0 J/s  Q_nominal_specify=off  Q_nominal_unit=W  Q_nominal_value=1
  Evaporator Pipe : refrigeration_lib/Pipe  L=evaporator_length m  S=pi*pipe_diameter^2/4 m^2  Dh=pipe_diameter m  fs=64  La=0.1*evaporator_length m  eps=15e-6 m  Re_lam=2000  Re_tur=4000  J_smooth=5 kg/m^2/s  p_0=charge_pressure MPa  T_0=-1 K  x_0=initial_quality  mdot_A_specify=off  mdot_A_priority=High  mdot_A=0 kg/s  mdot_A_nominal_specify=off  mdot_A_nominal_unit=kg/s  mdot_A_nominal_value=1  mdot_B_specify=off  mdot_B_priority=High  mdot_B=0 kg/s  mdot_B_nominal_specify=off  mdot_B_nominal_unit=kg/s  mdot_B_nominal_value=1  phi_A_specify=off  phi_A_priority=High  phi_A=0 kW  phi_A_nominal_specify=off  phi_A_nominal_unit=kW  phi_A_nominal_value=1  phi_B_specify=off  phi_B_priority=High  phi_B=0 kW  phi_B_nominal_specify=off  phi_B_nominal_unit=kW  phi_B_nominal_value=1  v_A_specify=off  v_A_priority=High  v_A=0.230606289431 m^3/kg  v_A_nominal_specify=off  v_A_nominal_unit=m^3/kg  v_A_nominal_value=1  v_B_specify=off  v_B_priority=High  v_B=0.230606289431 m^3/kg  v_B_nominal_specify=off  v_B_nominal_unit=m^3/kg  v_B_nominal_value=1  p_I_specify=off  p_I_priority=High  p_I=0.101325 MPa  p_I_nominal_specify=off  p_I_nominal_unit=MPa  p_I_nominal_value=1  u_I_specify=off  u_I_priority=High  u_I=396.921741345 kJ/kg  u_I_nominal_specify=off  u_I_nominal_unit=kJ/kg  u_I_nominal_value=1  v_I_specify=off  v_I_priority=High  v_I=0.230606289431 m^3/kg  v_I_nominal_specify=off  v_I_nominal_unit=m^3/kg  v_I_nominal_value=1  q_T_specify=off  q_T_priority=High  q_T=0 kW  q_T_nominal_specify=off  q_T_nominal_unit=kW  q_T_nominal_value=1  Ff_A_specify=off  Ff_A_priority=High  Ff_A=0 N  Ff_A_nominal_specify=off  Ff_A_nominal_unit=N  Ff_A_nominal_value=1  Ff_B_specify=off  Ff_B_priority=High  Ff_B=0 N  Ff_B_nominal_specify=off  Ff_B_nominal_unit=N  Ff_B_nominal_value=1  ev_I_specify=off  ev_I_priority=High  ev_I=1.7212095226213e+3 kJ/m^3  ev_I_nominal_specify=off  ev_I_nominal_unit=kJ/m^3  ev_I_nominal_value=1  mdot_I_specify=off  mdot_I_priority=High  mdot_I=0 kg/s  mdot_I_nominal_specify=off  mdot_I_nominal_unit=kg/s  mdot_I_nominal_value=1  Nu_I_specify=off  Nu_I_priority=High  Nu_I=0  Nu_I_nominal_specify=off  Nu_I_nominal_unit=1  Nu_I_nominal_value=1
      settings: InternalSimscapePortConfiguration="{\"Bottom\":[],\"Left\":[{\"id\":\"A\",\"label\":\"A\",\"type\":\"refrigeration.refrigeration\"},{\"id\":\"T\",\"label\":\"T\",\"type\":\"foundation.thermal.thermal\"}],\"Right\":[{\"id\":\"B\",\"label\":\"B\",\"type\":\"refrigeration.refrigeration\"}],\"Top\":[]}"
  A : PMIOPort  Side=Left
  B : PMIOPort  Port=2  Side=Right
  T : PMIOPort  Port=3  Side=Right
  connections:
  Evaporator Conduction/RConn1 -- T/RConn1
  Evaporator Copper/LConn1 -- Evaporator Pipe/LConn2 -- Evaporator Conduction/LConn1
  Evaporator Pipe/RConn1 -- B/RConn1
  Evaporator Pipe/LConn1 -- A/RConn1

== system V.1.0.SystemsmModelling/Air Conditioning System/Air Conditioner Model7/Expansion Valve ==
  Controlled Local Restriction : refrigeration_lib/Controlled Local Restriction  Cd=0.7  L=0.1 m  S=pi*pipe_diameter^2/4 m^2
      settings: InternalSimscapePortConfiguration="{\"Bottom\":[],\"Left\":[{\"id\":\"A\",\"label\":\"A\",\"type\":\"refrigeration.refrigeration\"},{\"id\":\"Sr\",\"label\":\"S\",\"type\":\"input\"}],\"Right\":[{\"id\":\"B\",\"label\":\"B\",\"type\":\"refrigeration.refrigeration\"}],\"Top\":[]}"
  Cycle Sensor 4 : Subsystem
  Mass Flow Sensor : Subsystem
  Valve Control : Subsystem
  A : PMIOPort  Side=Left
  B : PMIOPort  Port=2  Side=Right
  connections:
  B/RConn1 -- Cycle Sensor 4/LConn1 -- Mass Flow Sensor/RConn1
  Controlled Local Restriction/LConn1 -- A/RConn1
  Controlled Local Restriction/RConn1 -- Mass Flow Sensor/LConn1
  Controlled Local Restriction/LConn2 -- Valve Control/LConn1
  Cycle Sensor 4/RConn1 -- Valve Control/RConn1

== system V.1.0.SystemsmModelling/Air Conditioning System/Air Conditioner Model7/Plot Properties ==

== system V.1.0.SystemsmModelling/Air Conditioning System/Air Conditioner Model7/Refrigerator Compartment ==
  Environment Temperature : Subsystem
  Evaporator Convection : fl_lib/Thermal/Thermal Elements/Convective Heat Transfer  area=interior_surface_area m^2  heat_tr_coeff=natural_convection_coefficient W/(m^2 * K)  T_specify=off  T_priority=High  T=0 K  T_nominal_specify=off  T_nominal_unit=K  T_nominal_value=1  Q_specify=off  Q_priority=High  Q=0 J/s  Q_nominal_specify=off  Q_nominal_unit=W  Q_nominal_value=1
  Heat Flow Sensor : Subsystem
  Polyurethane Foam Conduction : fl_lib/Thermal/Thermal Elements/Conductive Heat Transfer  area=interior_surface_area m^2  thickness=foam_thickness m  th_cond=foam_conductivity W/(m*K)  T_specify=off  T_priority=High  T=0 K  T_nominal_specify=off  T_nominal_unit=K  T_nominal_value=1  Q_specify=off  Q_priority=High  Q=0 J/s  Q_nominal_specify=off  Q_nominal_unit=W  Q_nominal_value=1
  Refrigerator Convection Exterior : fl_lib/Thermal/Thermal Elements/Convective Heat Transfer  area=exterior_surface_area m^2  heat_tr_coeff=natural_convection_coefficient W/(m^2 * K)  T_specify=off  T_priority=High  T=0 K  T_nominal_specify=off  T_nominal_unit=K  T_nominal_value=1  Q_specify=off  Q_priority=High  Q=0 J/s  Q_nominal_specify=off  Q_nominal_unit=W  Q_nominal_value=1
  Refrigerator Convection Interior : fl_lib/Thermal/Thermal Elements/Convective Heat Transfer  area=interior_surface_area m^2  heat_tr_coeff=natural_convection_coefficient W/(m^2 * K)  T_specify=off  T_priority=High  T=0 K  T_nominal_specify=off  T_nominal_unit=K  T_nominal_value=1  Q_specify=off  Q_priority=High  Q=0 J/s  Q_nominal_specify=off  Q_nominal_unit=W  Q_nominal_value=1
  Temperature Sensor : Subsystem
  T : PMIOPort  Side=Left
  Air : PMIOPort  Port=2  Side=Left
  S : Outport
  wires:
  Temperature Sensor/1(T) -> S/1
  connections:
  Evaporator Convection/LConn1 -- Heat Flow Sensor/RConn1
  T/RConn1 -- Heat Flow Sensor/LConn1
  Refrigerator Convection Exterior/RConn1 -- Environment Temperature/LConn1
  Refrigerator Convection Interior/LConn1 -- Evaporator Convection/RConn1 -- Temperature Sensor/LConn1 -- Air/RConn1
  Refrigerator Convection Interior/RConn1 -- Polyurethane Foam Conduction/LConn1
  Polyurethane Foam Conduction/RConn1 -- Refrigerator Convection Exterior/LConn1

== system V.1.0.SystemsmModelling/Air Conditioning System/Air Conditioner Model8/Compressor ==
  On : Inport
  Commanded Mass Flow Rate : Gain  Gain=commanded_mass_flow
  Compressor Lag : TransferFcn  Numerator=[(9/compressor_time_constant)^2]  Denominator=[1, 2*(9/compressor_time_constant), (9/compressor_time_constant)^2]
  Controlled Mass Flow Rate Source : refrigeration_lib/Controlled Mass Flow Rate Source  S=pi*pipe_diameter^2/4 m^2  L=0.1 m  mdot_specify=off  mdot_priority=High  mdot=0 kg/s  mdot_nominal_specify=off  mdot_nominal_unit=kg/s  mdot_nominal_value=1  phi_A_specify=off  phi_A_priority=High  phi_A=0 kW  phi_A_nominal_specify=off  phi_A_nominal_unit=kW  phi_A_nominal_value=1  phi_B_specify=off  phi_B_priority=High  phi_B=0 kW  phi_B_nominal_specify=off  phi_B_nominal_unit=kW  phi_B_nominal_value=1  u_AI_specify=off  u_AI_priority=High  u_AI=396.921741345 kJ/kg  u_AI_nominal_specify=off  u_AI_nominal_unit=kJ/kg  u_AI_nominal_value=1  v_A_specify=off  v_A_priority=High  v_A=0.230606289431 m^3/kg  v_A_nominal_specify=off  v_A_nominal_unit=m^3/kg  v_A_nominal_value=1  u_BI_specify=off  u_BI_priority=High  u_BI=396.921741345 kJ/kg  u_BI_nominal_specify=off  u_BI_nominal_unit=kJ/kg  u_BI_nominal_value=1  v_B_specify=off  v_B_priority=High  v_B=0.230606289431 m^3/kg  v_B_nominal_specify=off  v_B_nominal_unit=m^3/kg  v_B_nominal_value=1  u_2_specify=off  u_2_priority=High  u_2=396.921741345 kJ/kg  u_2_nominal_specify=off  u_2_nominal_unit=kJ/kg  u_2_nominal_value=1  u_3_specify=off  u_3_priority=High  u_3=396.921741345 kJ/kg  u_3_nominal_specify=off  u_3_nominal_unit=kJ/kg  u_3_nominal_value=1
      settings: InternalSimscapePortConfiguration="{\"Bottom\":[],\"Left\":[{\"id\":\"A\",\"label\":\"A\",\"type\":\"refrigeration.refrigeration\"},{\"id\":\"M\",\"label\":\"M\",\"type\":\"input\"}],\"Right\":[{\"id\":\"B\",\"label\":\"B\",\"type\":\"refrigeration.refrigeration\"},{\"id\":\"W\",\"label\":\"W\",\"type\":\"output\"}],\"Top\":[]}"
  Simulink-PS Converter : nesl_utility/Simulink-PS Converter  PhysicalDomain=network_engine_domain  SubClassName=ps_input  LeftPortType=input  RightPortType=output  PseudoPeriodic=off  Frequencies=[]  NoiseDistribution=none  NoiseParameters=[]  Unit=kg/s  AffineConversion=off  FilteringAndDerivatives=zero  SimscapeFilterOrder=1  InputFilterTimeConstant=0.001  UdotUserProvided=1
  B : PMIOPort  Side=Right
  A : PMIOPort  Port=2  Side=Left
  wires:
  Compressor Lag/1 -> Simulink-PS Converter/1
  Commanded Mass Flow Rate/1 -> Compressor Lag/1
  On/1 -> Commanded Mass Flow Rate/1
  connections:
  Controlled Mass Flow Rate Source/RConn1 -- B/RConn1
  Controlled Mass Flow Rate Source/LConn2 -- Simulink-PS Converter/RConn1
  A/RConn1 -- Controlled Mass Flow Rate Source/LConn1

== system V.1.0.SystemsmModelling/Air Conditioning System/Air Conditioner Model8/Condenser ==
  Condenser Conduction : fl_lib/Thermal/Thermal Elements/Conductive Heat Transfer  area=pi*pipe_diameter*condenser_length m^2  thickness=pipe_thickness m  th_cond=copper_conductivity W/(m*K)  T_specify=off  T_priority=High  T=0 K  T_nominal_specify=off  T_nominal_unit=K  T_nominal_value=1  Q_specify=off  Q_priority=High  Q=0 J/s  Q_nominal_specify=off  Q_nominal_unit=W  Q_nominal_value=1
  Condenser Copper : fl_lib/Thermal/Thermal Elements/Thermal Mass  mass=pi*pipe_diameter*condenser_length*pipe_thickness*copper_density kg  sp_heat=copper_specific_heat J/kg/K  T_specify=on  T_priority=High  T=environment_temperature K  T_nominal_specify=off  T_nominal_unit=K  T_nominal_value=1  Q_specify=off  Q_priority=High  Q=0 J/s  Q_nominal_specify=off  Q_nominal_unit=W  Q_nominal_value=1
  Condenser Pipe : refrigeration_lib/Pipe  L=condenser_length m  S=pi*pipe_diameter^2/4 m^2  Dh=pipe_diameter m  fs=64  La=0.1*condenser_length m  eps=15e-6 m  Re_lam=2000  Re_tur=4000  J_smooth=5 kg/m^2/s  p_0=charge_pressure MPa  T_0=-1 K  x_0=initial_quality  mdot_A_specify=off  mdot_A_priority=High  mdot_A=0 kg/s  mdot_A_nominal_specify=off  mdot_A_nominal_unit=kg/s  mdot_A_nominal_value=1  mdot_B_specify=off  mdot_B_priority=High  mdot_B=0 kg/s  mdot_B_nominal_specify=off  mdot_B_nominal_unit=kg/s  mdot_B_nominal_value=1  phi_A_specify=off  phi_A_priority=High  phi_A=0 kW  phi_A_nominal_specify=off  phi_A_nominal_unit=kW  phi_A_nominal_value=1  phi_B_specify=off  phi_B_priority=High  phi_B=0 kW  phi_B_nominal_specify=off  phi_B_nominal_unit=kW  phi_B_nominal_value=1  v_A_specify=off  v_A_priority=High  v_A=0.230606289431 m^3/kg  v_A_nominal_specify=off  v_A_nominal_unit=m^3/kg  v_A_nominal_value=1  v_B_specify=off  v_B_priority=High  v_B=0.230606289431 m^3/kg  v_B_nominal_specify=off  v_B_nominal_unit=m^3/kg  v_B_nominal_value=1  p_I_specify=off  p_I_priority=High  p_I=0.101325 MPa  p_I_nominal_specify=off  p_I_nominal_unit=MPa  p_I_nominal_value=1  u_I_specify=off  u_I_priority=High  u_I=396.921741345 kJ/kg  u_I_nominal_specify=off  u_I_nominal_unit=kJ/kg  u_I_nominal_value=1  v_I_specify=off  v_I_priority=High  v_I=0.230606289431 m^3/kg  v_I_nominal_specify=off  v_I_nominal_unit=m^3/kg  v_I_nominal_value=1  q_T_specify=off  q_T_priority=High  q_T=0 kW  q_T_nominal_specify=off  q_T_nominal_unit=kW  q_T_nominal_value=1  Ff_A_specify=off  Ff_A_priority=High  Ff_A=0 N  Ff_A_nominal_specify=off  Ff_A_nominal_unit=N  Ff_A_nominal_value=1  Ff_B_specify=off  Ff_B_priority=High  Ff_B=0 N  Ff_B_nominal_specify=off  Ff_B_nominal_unit=N  Ff_B_nominal_value=1  ev_I_specify=off  ev_I_priority=High  ev_I=1.7212095226213e+3 kJ/m^3  ev_I_nominal_specify=off  ev_I_nominal_unit=kJ/m^3  ev_I_nominal_value=1  mdot_I_specify=off  mdot_I_priority=High  mdot_I=0 kg/s  mdot_I_nominal_specify=off  mdot_I_nominal_unit=kg/s  mdot_I_nominal_value=1  Nu_I_specify=off  Nu_I_priority=High  Nu_I=0  Nu_I_nominal_specify=off  Nu_I_nominal_unit=1  Nu_I_nominal_value=1
      settings: InternalSimscapePortConfiguration="{\"Bottom\":[],\"Left\":[{\"id\":\"A\",\"label\":\"A\",\"type\":\"refrigeration.refrigeration\"},{\"id\":\"T\",\"label\":\"T\",\"type\":\"foundation.thermal.thermal\"}],\"Right\":[{\"id\":\"B\",\"label\":\"B\",\"type\":\"refrigeration.refrigeration\"}],\"Top\":[]}"
  T : PMIOPort  Side=Left
  B : PMIOPort  Port=2  Side=Left
  A : PMIOPort  Port=3  Side=Right
  connections:
  Condenser Conduction/LConn1 -- Condenser Pipe/LConn2 -- Condenser Copper/LConn1
  T/RConn1 -- Condenser Conduction/RConn1
  B/RConn1 -- Condenser Pipe/RConn1
  Condenser Pipe/LConn1 -- A/RConn1
